simulink model "raspi_test"  (R2018b)
settings: Solver=FixedStepAuto  StartTime=0.0  StopTime=inf  RelTol=1e-3  EnableMultiTasking=on
libraries: embdlinuxlib x2, raspberrypilib x1
settings Model: SimulationMode=external  EnablePacing=on  ExtModeTrigDuration=2  Creator=benkl  LastModifiedBy=benkl
settings SolverCC: PositivePriorityOrder=on  AutoInsertRateTranBlk=on
settings OptimizationCC: EnhancedBackFolding=on  PassReuseOutputArgsAs=Individual arguments  MaxStackSize=64  OptimizeBlockOrder=speed  DifferentSizesBufferReuse=on  OptimizationCustomize=off
settings DebuggingCC: ParameterTunabilityLossMsg=error
settings HardwareCC: ProdBitPerPointer=32  ProdBitPerSizeT=32  ProdBitPerPtrDiffT=32  ProdLargestAtomicInteger=Long  ProdLargestAtomicFloat=Double  ProdWordSize=32  ProdHWDeviceType=ARM Compatible->ARM Cortex
settings SFSimCC: MATLABDynamicMemAlloc=off
settings RTWCC: SystemTargetFile=ert.tlc  HardwareBoard=Raspberry Pi  TLCOptions="-aInlineSetEventsForThisBaseRateFcn=TLC_FALSE -aSuppressMultiTaskScheduler=TLC_FALSE  -aRateBasedStepFcn=0"  TemplateMakefile=ert_default_tmf  GenerateReport=on  Toolchain=GNU GCC Raspberry Pi  BuildConfiguration=Faster Runs  IncludeHyperlinkInReport=on  LaunchReport=on  GenerateTraceInfo=on  GenerateTraceReport=on  GenerateTraceReportSl=on  GenerateTraceReportSf=on  GenerateTraceReportEml=on
settings CodeAppCC: ForceParamTrailComments=on  IgnoreCustomStorageClasses=off  OperatorAnnotations=on  SimulinkDataObjDesc=on  SFDataObjDesc=on  InsertBlockDesc=on
settings ERTTargetCC: SupportContinuousTime=on  SupportVariableSizeSignals=on

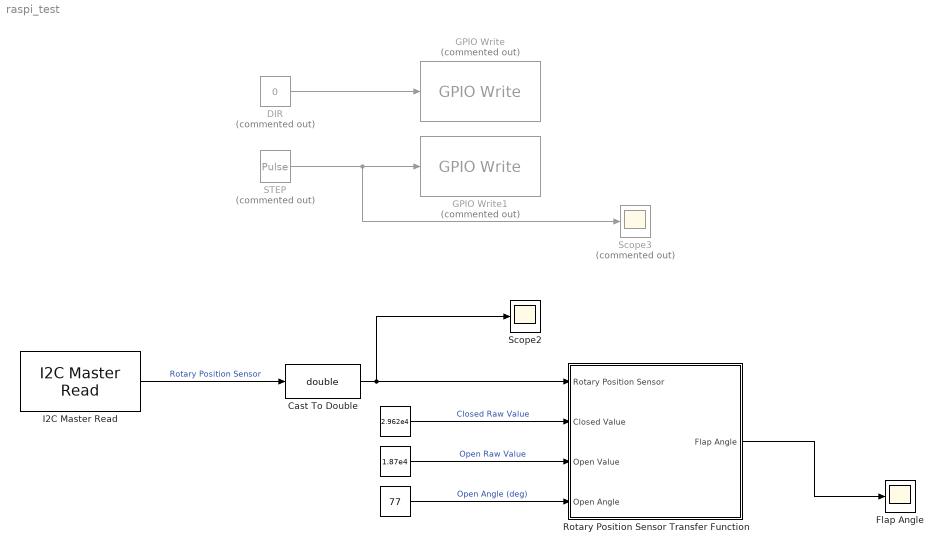
== system raspi_test ==
  " " : Constant  Value=2.962e4
  "  " : Constant  Value=77
  " " : Constant  Value=1.87e4
  Cast To Double : DataTypeConversion  OutDataTypeStr=double
  DIR : Constant  Commented=on  Value=0
  Flap Angle : Scope
  GPIO Write : embdlinuxlib/GPIO Write  Commented=on  board=Model B+  gpio=21  direction=Output  blockPlatform=Raspberry Pi
      settings: SourceProductName=Simulink Support Package for Raspberry Pi Hardware  SourceProductBaseCode=RASPPI
  GPIO Write1 : embdlinuxlib/GPIO Write  Commented=on  board=Model B+  gpio=20  direction=Output  blockPlatform=Raspberry Pi
      settings: SourceProductName=Simulink Support Package for Raspberry Pi Hardware  SourceProductBaseCode=RASPPI
  I2C Master Read : raspberrypilib/I2C Master Read  BoardProperty=Pi 3 Model B+  Mode=Master  SlaveAddress=72  SlaveByteOrder=BigEndian  Direction=Receiver  RegisterAddressMode=on  RegisterAddress=0  SlaveDataType=int16  DataLength=1  NoAck=off  RepeatedStart=off  OutputStatus=off  SampleTime=0.1
      settings: SourceProductName=Simulink Support Package for Raspberry Pi Hardware  SourceProductBaseCode=RASPPI
  Rotary Position Sensor Transfer Function : Subsystem
  STEP : DiscretePulseGenerator  Commented=on  PulseType=Time based  Period=0.01  PulseWidth=50
  Scope2 : Scope
  Scope3 : Scope  Commented=on
  wires:
  " "/1 -> Rotary Position Sensor Transfer Function/2(Closed Value)  "Closed Raw Value"
  " "/1 -> Rotary Position Sensor Transfer Function/3(Open Value)  "Open Raw Value"
  Rotary Position Sensor Transfer Function/1(Flap Angle) -> Flap Angle/1
  I2C Master Read/1 -> Cast To Double/1  "Rotary Position Sensor"
  "  "/1 -> Rotary Position Sensor Transfer Function/4(Open Angle)  "Open Angle (deg)"
  DIR/1 -> GPIO Write/1
  STEP/1 -> Scope3/1, GPIO Write1/1
  Cast To Double/1 -> Scope2/1, Rotary Position Sensor Transfer Function/1(Rotary Position Sensor)

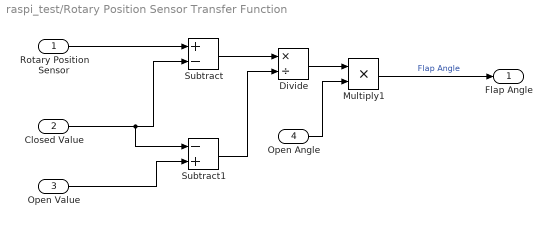
== system raspi_test/Rotary Position Sensor Transfer Function ==
  Rotary Position Sensor : Inport
  Closed Value : Inport  Port=2
  Open Value : Inport  Port=3
  Open Angle : Inport  Port=4
  Divide : Product  Inputs=*/
  Multiply1 : Product
  Subtract : Sum  Inputs=+-
  Subtract1 : Sum  Inputs=-+
  Flap Angle : Outport
  wires:
  Subtract/1 -> Divide/1
  Closed Value/1 -> Subtract1/1, Subtract/2
  Divide/1 -> Multiply1/1
  Open Angle/1 -> Multiply1/2
  Subtract1/1 -> Divide/2
  Rotary Position Sensor/1 -> Subtract/1
  Open Value/1 -> Subtract1/2
  Multiply1/1 -> Flap Angle/1  "Flap Angle"
